simulink model "sampleModel1943"  (R2023a)
settings: Solver=VariableStepAuto  StartTime=0.0  StopTime=10.0  RelTol=1e-3
libraries: hdlsllib x6, simulink x2
settings Model: Creator=user1  LastModifiedBy=user1

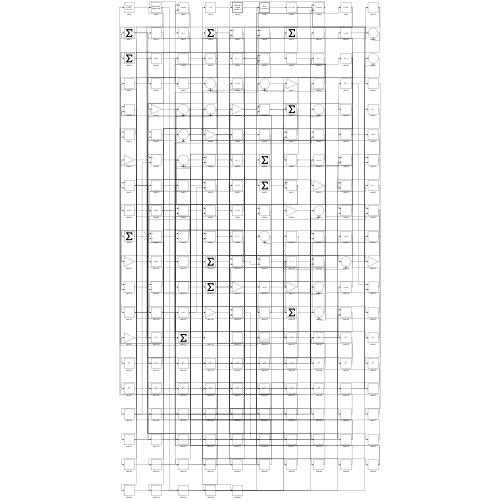
[thumbnail: Simulink's stored preview of the top-level diagram]
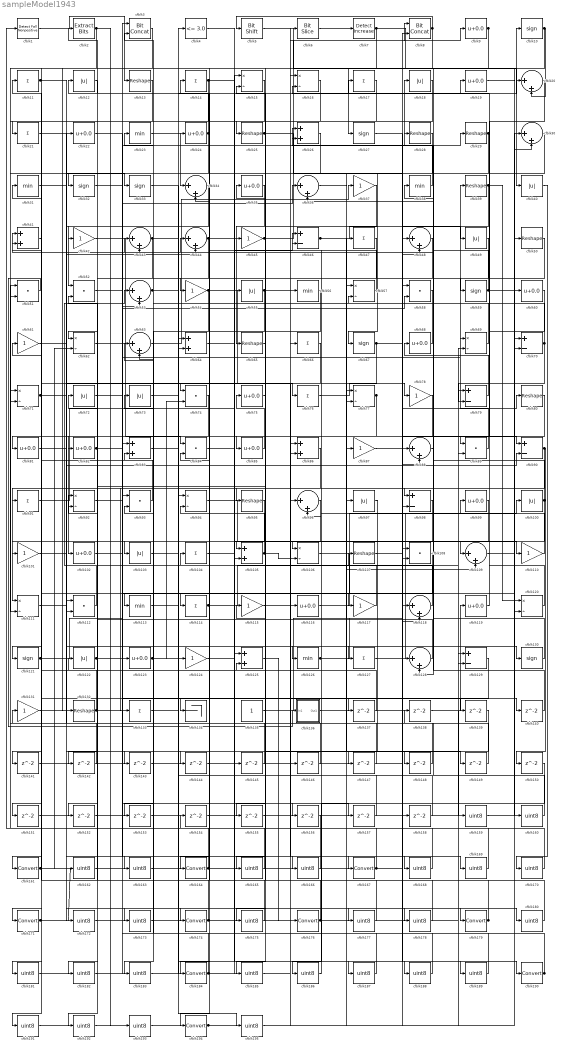
== system sampleModel1943 ==
  cfblk1 : hdlsllib/Logic and Bit Operations/Detect Fall Nonpositive  vinit=0  OutDataTypeStr=boolean
  cfblk{10,27,32..33,59,67,121,130} (8 alike) : Signum
  cfblk{12,18,40,49,55,72..73,97,100,103,122} (11 alike) : Abs  SaturateOnIntegerOverflow=off
  cfblk{37,42,45,54,61,78,87,101,110,115,117,124,131} (13 alike) : Gain
  cfblk{9,19,22,24,35,60,68,75,81..82,85,99,102,116,119,123} (16 alike) : Bias  Bias=0.0  SaturateOnIntegerOverflow=off
  cfblk{11,14,17,21,47,66,76,91,104,114,127,133} (12 alike) : Sum  Inputs=+
  cfblk{26,41,64,83,86,105,125} (7 alike) : Sum
  cfblk{15..16,57,62,69,71,77,92,94,106,111,120} (12 alike) : Product  Inputs=*/  RndMeth=Zero  SaturateOnIntegerOverflow=on
  cfblk{13,25,28..29,39,50,65,80,95,107,132} (11 alike) : Reshape
  cfblk{51..52,58,74,84,89,93,108,112} (9 alike) : DotProduct  OutDataTypeStr=Inherit: Inherit via internal rule
  cfblk{20,30,34,36,43..44,48,53,63,88,96,109,118,128} (14 alike) : Sum  Inputs=|++
  cfblk{23,31,38,56,113,126} (6 alike) : MinMax
  cfblk{46,70,79,90,98,129} (6 alike) : Sum  Inputs=+-
  cfblk134 : Terminator
  cfblk135 : Constant  SampleTime=-1
  cfblk136 : Subsystem
      settings: LibrarySourceBlock=|
      | hdlsllib/Ports &
      | Subsystems/Subsystem
  cfblk{137..158} (22 alike) : Delay  SampleTime=1
  cfblk{159..160,162..163,165..166,168..170,172..173,175,177..178,180..183,185..189,191..193,195} (27 alike) : DataTypeConversion  OutDataTypeStr=uint8  SaturateOnIntegerOverflow=off  RndMeth=Floor
  cfblk{161,164,167,171,174,176,179,184,190,194} (10 alike) : DataTypeConversion  SaturateOnIntegerOverflow=off  RndMeth=Floor
  cfblk2 : simulink/Logic and Bit Operations/Extract Bits  bitsToExtract=Upper half  numBits=8  bitIdxRange=[0 7]  outScalingMode=Preserve fixed-point scaling
      settings: LibrarySourceBlock=|
      | hdlsllib/Logic and Bit
      | Operations/Extract Bits
  cfblk3 : hdlsllib/Logic and Bit Operations/Bit Concat  numInputs=2
  cfblk4 : hdlsllib/Logic and Bit Operations/Compare To Constant  relop=<=  const=3.0  OutDataTypeStr=boolean
  cfblk5 : hdlsllib/Logic and Bit Operations/Bit Shift  mode=Shift Left Logical  N=0
  cfblk6 : hdlsllib/Logic and Bit Operations/Bit Slice  lidx=7  ridx=0
  cfblk7 : simulink/Logic and Bit Operations/Detect Increase  vinit=0.0  OutDataTypeStr=boolean
      settings: LibrarySourceBlock=|
      | hdlsllib/Logic and Bit
      | Operations/Detect
      | Increase
  cfblk8 : hdlsllib/Logic and Bit Operations/Bit Concat  numInputs=2
  wires:
  cfblk74/1 -> cfblk102/1
  cfblk42/1 -> cfblk84/1
  cfblk69/1 -> cfblk52/1
  cfblk60/1 -> cfblk68/1
  cfblk85/1 -> cfblk75/1
  cfblk95/1 -> cfblk103/1
  cfblk88/1 -> cfblk38/1
  cfblk30/1 -> cfblk32/1
  cfblk112/1 -> cfblk53/1
  cfblk68/1 -> cfblk12/1
  cfblk2/1 -> cfblk132/1, cfblk193/1
  cfblk90/1 -> cfblk133/1, cfblk150/1
  cfblk75/1 -> cfblk131/1
  cfblk25/1 -> cfblk8/1, cfblk48/2
  cfblk31/1 -> cfblk33/1
  cfblk38/1 -> cfblk18/1
  cfblk87/1 -> cfblk190/1
  cfblk78/1 -> cfblk81/1
  cfblk115/1 -> cfblk167/1
  cfblk127/1 -> cfblk100/1
  cfblk67/1 -> cfblk109/1, cfblk151/1
  cfblk89/1 -> cfblk39/1
  cfblk94/1 -> cfblk106/1
  cfblk44/1 -> cfblk142/1, cfblk168/1
  cfblk54/1 -> cfblk116/1, cfblk46/1, cfblk113/1, cfblk178/1
  cfblk136/1(Out1) -> cfblk119/1
  cfblk120/1 -> cfblk16/2
  cfblk35/1 -> cfblk65/1
  cfblk76/1 -> cfblk78/1
  cfblk128/1 -> cfblk72/1
  cfblk5/1 -> cfblk40/1
  cfblk80/1 -> cfblk134/1
  cfblk8/1 -> cfblk5/1, cfblk185/1
  cfblk45/1 -> cfblk10/1, cfblk9/1
  cfblk111/1 -> cfblk22/1
  cfblk26/1 -> cfblk105/1
  cfblk77/1 -> cfblk101/1, cfblk153/1
  cfblk63/1 -> cfblk37/1
  cfblk123/1 -> cfblk74/2, cfblk157/1
  cfblk4/1 -> cfblk110/1
  cfblk79/1 -> cfblk28/1
  cfblk55/1 -> cfblk6/1, cfblk183/1
  cfblk59/1 -> cfblk30/2, cfblk36/2
  cfblk116/1 -> cfblk99/1
  cfblk125/1 -> cfblk176/1
  cfblk119/1 -> cfblk19/1
  cfblk11/1 -> cfblk143/1, cfblk144/1
  cfblk135/1 -> cfblk80/1
  cfblk43/1 -> cfblk62/1, cfblk188/1
  cfblk100/1 -> cfblk41/1, cfblk114/1
  cfblk23/1 -> cfblk34/1
  cfblk110/1 -> cfblk44/1
  cfblk29/1 -> cfblk89/1, cfblk67/1, cfblk77/2
  cfblk27/1 -> cfblk90/1
  cfblk49/1 -> cfblk98/1
  cfblk132/1 -> cfblk31/1, cfblk36/1
  cfblk51/1 -> cfblk136/1(In1)
  cfblk9/1 -> cfblk54/1, cfblk128/2
  cfblk114/1 -> cfblk89/2, cfblk77/1
  cfblk39/1 -> cfblk98/2, cfblk120/1
  cfblk62/1 -> cfblk124/1
  cfblk48/1 -> cfblk85/1
  cfblk103/1 -> cfblk117/1
  cfblk122/1 -> cfblk139/1, cfblk140/1
  cfblk91/1 -> cfblk55/1
  cfblk10/1 -> cfblk27/1, cfblk20/2
  cfblk102/1 -> cfblk130/1
  cfblk20/1 -> cfblk59/1
  cfblk1/1 -> cfblk13/1
  cfblk130/1 -> cfblk43/1
  cfblk17/1 -> cfblk121/1
  cfblk70/1 -> cfblk23/1, cfblk79/2
  cfblk24/1 -> cfblk2/1, cfblk191/1
  cfblk84/1 -> cfblk26/1
  cfblk61/1 -> cfblk174/1
  cfblk86/1 -> cfblk111/1
  cfblk3/1 -> cfblk71/2
  cfblk106/1 -> cfblk118/2
  cfblk6/1 -> cfblk7/1
  cfblk53/1 -> cfblk126/1, cfblk17/1
  cfblk108/1 -> cfblk161/1
  cfblk105/1 -> cfblk94/2, cfblk106/2
  cfblk13/1 -> cfblk42/1
  cfblk96/1 -> cfblk184/1
  cfblk32/1 -> cfblk29/1
  cfblk126/1 -> cfblk88/1, cfblk46/2
  cfblk131/1 -> cfblk44/2
  cfblk121/1 -> cfblk43/2, cfblk90/2, cfblk127/1
  cfblk18/1 -> cfblk25/1
  cfblk28/1 -> cfblk51/2
  cfblk117/1 -> cfblk107/1
  cfblk64/1 -> cfblk179/1
  cfblk129/1 -> cfblk171/1
  cfblk71/1 -> cfblk76/1, cfblk163/1, cfblk173/1
  cfblk46/1 -> cfblk49/1, cfblk109/2
  cfblk34/1 -> cfblk112/2
  cfblk92/1 -> cfblk58/2
  cfblk82/1 -> cfblk69/1, cfblk120/2
  cfblk58/1 -> cfblk57/2
  cfblk93/1 -> cfblk41/2
  cfblk65/1 -> cfblk95/1
  cfblk22/1 -> cfblk74/1
  cfblk15/1 -> cfblk164/1
  cfblk118/1 -> cfblk92/1
  cfblk50/1 -> cfblk82/1
  cfblk133/1 -> cfblk24/1
  cfblk56/1 -> cfblk194/1
  cfblk73/1 -> cfblk4/1
  cfblk16/1 -> cfblk111/2
  cfblk57/1 -> cfblk14/1
  cfblk109/1 -> cfblk60/1
  cfblk14/1 -> cfblk91/1, cfblk137/1
  cfblk7/1 -> cfblk70/2, cfblk20/1, cfblk21/1
  cfblk137/1 -> cfblk92/2
  cfblk140/1 -> cfblk26/2
  cfblk41/1 -> cfblk141/1
  cfblk141/1 -> cfblk86/1
  cfblk142/1 -> cfblk71/1
  cfblk143/1 -> cfblk118/1
  cfblk144/1 -> cfblk8/2
  cfblk145/1 -> cfblk3/1
  cfblk146/1 -> cfblk84/2
  cfblk97/1 -> cfblk147/1
  cfblk147/1 -> cfblk112/1
  cfblk33/1 -> cfblk148/1
  cfblk148/1 -> cfblk34/2
  cfblk36/1 -> cfblk149/1
  cfblk149/1 -> cfblk58/1
  cfblk151/1 -> cfblk53/2
  cfblk12/1 -> cfblk152/1
  cfblk152/1 -> cfblk30/1
  cfblk153/1 -> cfblk57/1
  cfblk154/1 -> cfblk105/2
  cfblk37/1 -> cfblk155/1
  cfblk155/1 -> cfblk88/2
  cfblk72/1 -> cfblk156/1
  cfblk156/1 -> cfblk1/1
  cfblk157/1 -> cfblk94/1
  cfblk107/1 -> cfblk158/1
  cfblk158/1 -> cfblk35/1
  cfblk138/1 -> cfblk159/1
  cfblk159/1 -> cfblk70/1
  cfblk19/1 -> cfblk160/1
  cfblk160/1 -> cfblk138/1
  cfblk161/1 -> cfblk146/1, cfblk145/1, cfblk62/2
  cfblk162/1 -> cfblk108/1
  cfblk163/1 -> cfblk108/2
  cfblk164/1 -> cfblk86/2, cfblk122/1
  cfblk139/1 -> cfblk165/1
  cfblk165/1 -> cfblk15/1
  cfblk52/1 -> cfblk166/1
  cfblk166/1 -> cfblk15/2
  cfblk167/1 -> cfblk11/1, cfblk51/1
  cfblk168/1 -> cfblk115/1
  cfblk104/1 -> cfblk169/1
  cfblk169/1 -> cfblk79/1
  cfblk40/1 -> cfblk170/1
  cfblk170/1 -> cfblk104/1
  cfblk171/1 -> cfblk162/1, cfblk97/1
  cfblk21/1 -> cfblk172/1
  cfblk172/1 -> cfblk129/1
  cfblk173/1 -> cfblk129/2
  cfblk174/1 -> cfblk48/1, cfblk63/1
  cfblk99/1 -> cfblk175/1
  cfblk175/1 -> cfblk61/1
  cfblk176/1 -> cfblk154/1, cfblk63/2
  cfblk101/1 -> cfblk177/1
  cfblk177/1 -> cfblk125/1
  cfblk178/1 -> cfblk125/2
  cfblk179/1 -> cfblk73/1, cfblk52/2
  cfblk81/1 -> cfblk180/1
  cfblk180/1 -> cfblk64/1
  cfblk98/1 -> cfblk181/1
  cfblk181/1 -> cfblk64/2
  cfblk66/1 -> cfblk182/1
  cfblk182/1 -> cfblk123/1
  cfblk183/1 -> cfblk66/1
  cfblk184/1 -> cfblk45/1, cfblk3/2
  cfblk185/1 -> cfblk96/1
  cfblk150/1 -> cfblk186/1
  cfblk186/1 -> cfblk96/2
  cfblk83/1 -> cfblk187/1
  cfblk187/1 -> cfblk93/1
  cfblk188/1 -> cfblk83/1
  cfblk124/1 -> cfblk189/1
  cfblk189/1 -> cfblk83/2
  cfblk190/1 -> cfblk93/2, cfblk16/1
  cfblk191/1 -> cfblk87/1
  cfblk47/1 -> cfblk192/1
  cfblk192/1 -> cfblk50/1
  cfblk193/1 -> cfblk47/1
  cfblk194/1 -> cfblk128/1, cfblk69/2
  cfblk113/1 -> cfblk195/1
  cfblk195/1 -> cfblk56/1

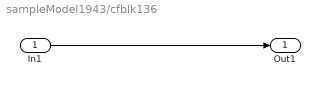
== system sampleModel1943/cfblk136 ==
  In1 : Inport
  Out1 : Outport
  wires:
  In1/1 -> Out1/1
